simulink model "a3"  (R2021a)
settings: Solver=ode23  StartTime=0.0  StopTime=5  RelTol=1e-3  EnableMultiTasking=on
undefined symbols (not defined in the file or in its folder): Ion, Lithium
libraries: spsCurrentMeasurementLib x25, spsVoltageMeasurementLib x19, spsSeriesRLCBranchLib x12, spsGroundLib x6, powerlib_extras x4, spsIGBTDiodeLib x3, dspsigops x3, spsPower3phInstantaneousLib x3, eeTotalHarmonicDistorsion x3, spsUniversalBridgeLib x2, spsBatteryLib x1, spsDiodeLib x1
(part 2 of 2)

== system a3/Control Algorithm/Subsystem2/Subsystem5 ==
  I : Inport
  Constant3 : Constant  Value=100
  Constant4 : Constant  Value=-98683.93
  Integrator3 : Integrator
  Integrator4 : Integrator
  Product6 : Product  RndMeth=Zero
  Product7 : Product  RndMeth=Zero
  Sum6 : Sum  Inputs=+-
  Sum7 : Sum
  Transfer Fcn : TransferFcn  Denominator=[2.65e-3 1]
  O : Outport
  wires:
  Integrator4/1 -> O/1, Product7/2, Sum6/2
  Sum6/1 -> Transfer Fcn/1
  Transfer Fcn/1 -> Product6/1
  Constant3/1 -> Product6/2
  Product6/1 -> Sum7/1
  Integrator3/1 -> Sum7/2
  Product7/1 -> Integrator3/1
  Constant4/1 -> Product7/1
  Sum7/1 -> Integrator4/1
  I/1 -> Sum6/1

== system a3/Control Algorithm/Subsystem2/Subsystem6 ==
  I : Inport
  Constant3 : Constant  Value=100
  Constant4 : Constant  Value=-98683.93
  Integrator3 : Integrator
  Integrator4 : Integrator
  Product6 : Product  RndMeth=Zero
  Product7 : Product  RndMeth=Zero
  Sum6 : Sum  Inputs=+-
  Sum7 : Sum
  Transfer Fcn : TransferFcn  Denominator=[2.65e-3 1]
  O : Outport
  wires:
  I/1 -> Sum6/1
  Sum7/1 -> Integrator4/1
  Constant4/1 -> Product7/1
  Product7/1 -> Integrator3/1
  Integrator3/1 -> Sum7/2
  Product6/1 -> Sum7/1
  Constant3/1 -> Product6/2
  Transfer Fcn/1 -> Product6/1
  Sum6/1 -> Transfer Fcn/1
  Integrator4/1 -> Sum6/2, Product7/2, O/1

== system a3/PV Array/PV Module1/Subsystem ==
  note: Delta T
  note: Io
  Add4 : Sum  Inputs=+-
  Add5 : Sum
  Add6 : Sum
  Add7 : Sum  Inputs=+-
  Constant8 : Constant
  Divide2 : Product  Inputs=**
  Divide4 : Product  Inputs=*/
  Math Function1 : Math  SignedPower=on  SaturateOnIntegerOverflow=on
  Product4 : Product  RndMeth=Zero
  Product5 : Product  RndMeth=Zero
  Out1 : Outport
  wires:
  [Vt1] -> Divide2/2
  Divide4/1 -> Out1/1
  Add7/1 -> Divide4/2
  Divide2/1 -> Math Function1/1
  Constant8/1 -> Add7/2
  Math Function1/1 -> Add7/1
  Add6/1 -> Divide2/1
  Product5/1 -> Add6/1
  [Kv] -> Product5/2
  [Vocn1] -> Add6/2
  [Tn] -> Add4/2
  Add5/1 -> Divide4/1
  [Iscn1] -> Add5/1
  Product4/1 -> Add5/2
  [Ki] -> Product4/1
  Add4/1 -> Product5/1, Product4/2
  [T1] -> Add4/1

== system a3/PV Array/PV Module1/Subsystem2 ==
  note: Ipv
  note: Delta T
  Add2 : Sum  Inputs=+-
  Add3 : Sum
  Divide1 : Product  Inputs=*/
  Product2 : Product  RndMeth=Zero
  Product3 : Product  RndMeth=Zero
  Out1 : Outport
  wires:
  [G1] -> Divide1/1
  [Gn] -> Divide1/2
  Divide1/1 -> Product3/2
  [Tn] -> Add2/2
  [T1] -> Add2/1
  Add2/1 -> Product2/2
  [Ki] -> Product2/1
  Product2/1 -> Add3/2
  [Ipvn1] -> Add3/1
  Add3/1 -> Product3/1
  Product3/1 -> Out1/1

== system a3/PV Array/PV Module1/Vt ==
  note: Ns
  note: K
  note: q
  note: a
  note: T1
  Constant1 : Constant  Value=54
  Constant3 : Constant  Value=1.3806503e-23
  Constant6 : Constant  Value=1.60217646e-19
  Divide2 : Product  Inputs=*/
  Divide3 : Product  Inputs=/*
  Divide4 : Product  Inputs=***
  Vt : Outport
  wires:
  Divide3/1 -> Divide2/1
  Divide4/1 -> Divide3/1
  [T1] -> Divide2/2
  Constant6/1 -> Divide3/2
  Constant3/1 -> Divide4/3
  Constant1/1 -> Divide4/2
  [a] -> Divide4/1
  Divide2/1 -> Vt/1

== matlab function a3/MPPT ==
  settings: updateMethod=DISCRETE  sampleTime=1e-4
  data: tv input; Ipvin input; Vpvin input; Ipvin1 input; Vpvin1 input; Vdcref output; Vdcrefold input
function Vdcref = fcn(tv,Ipvin,Vpvin,Ipvin1,Vpvin1,Vdcrefold)
%#codegen
delVdc=0.2;
a=10;
delVpv=Vpvin-Vpvin1;
delIpv=Ipvin-Ipvin1;
if(tv>=0.6)
if(delVpv==0)
    if(delIpv==0)
        Vdcrefnew=Vdcrefold;
    else
        if(delIpv>0)
            Vdcrefnew=Vdcrefold-(delIpv/delVpv)*a;
    else
        Vdcrefnew=Vdcrefold+(delIpv/delVpv)*a;
        end
    end
    else
        if(delIpv/delVpv==-Ipvin/Vpvin)
            Vdcrefnew=Vdcrefold;
        else
            if(delIpv/delVpv>-Ipvin/Vpvin)
                Vdcrefnew=Vdcrefold-(delIpv/delVpv)*a;
            else
                Vdcrefnew=Vdcrefold+(delIpv/delVpv)*a;
            end
        end
end
Vdcref=Vdcrefnew;
else
Vdcref=280;
end


%Vdcref=658;

== matlab function a3/Battery/MATLAB Function ==
  data: discharge input; y output; charge input; soc input; override input; midcontrol input
function y = fcn(discharge,charge,soc,override,midcontrol)

if(soc<8.995 && override==0)
    y = charge;
else
    if(soc<8.995 && override==1)
        y = discharge;
    else
        if(soc>9.005 && override==0)
        y = discharge; 
        else
           if(soc>9.005 && override==1)
             y = charge; 
           else
               if(midcontrol == 0)
                   y =charge;
               else
                   y = discharge;
               end
           end
        end
    end
end
